simulink model "test9_1"  (R2024a)
settings: Solver=FixedStepAuto  StartTime=0.0  StopTime=20  FixedStep=0.001  MaxStep=1e-2  RelTol=1e-3
libraries: fl_lib x14, nesl_utility x12, simulink x5, sdl_lib x4
settings Model: DataDictionary=test4.sldd  Creator=18311  LastModifiedBy=18311

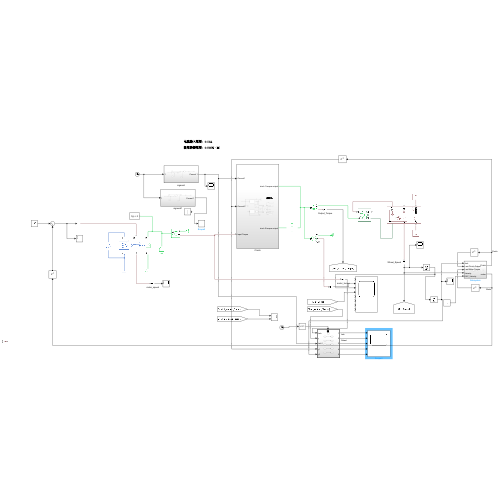
[thumbnail: Simulink's stored preview of the top-level diagram]
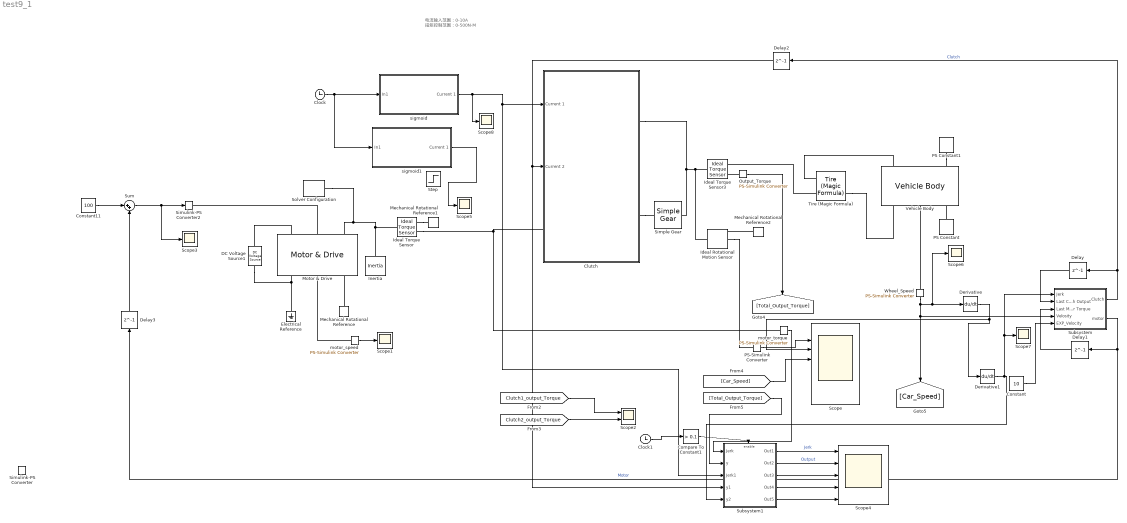
== system test9_1 ==
  note: 电流输入范围：0-10A
      | 扭矩控制范围：0-500N·M
  Clock : Clock
  Clock1 : Clock
  Clutch : Subsystem
  Compare To Constant1 : simulink/Logic and Bit Operations/Compare To Constant  relop=>  const=0.1  OutDataTypeStr=boolean
  Constant : Constant  Value=10
  Constant11 : Constant  Value=100
  DC Voltage Source1 : fl_lib/Electrical/Electrical Sources/DC Voltage Source  v0=220 V
  Delay{,1..3} (4 alike) : Delay  DelayLength=1  InitialCondition=0
  Derivative : Derivative
  Derivative1 : Derivative
  Electrical Reference : fl_lib/Electrical/Electrical Elements/Electrical Reference
  Ideal Rotational Motion Sensor : fl_lib/Mechanical/Mechanical Sensors/Ideal Rotational Motion Sensor  reference=foundation.enum.MeasurementReference.difference  acceleration_port=false  velocity_port=true  position_port=true  wrap_angle=false  offset=0 rad
  Ideal Torque Sensor : fl_lib/Mechanical/Mechanical Sensors/Ideal Torque Sensor
  Ideal Torque Sensor3 : fl_lib/Mechanical/Mechanical Sensors/Ideal Torque Sensor
  Inertia : fl_lib/Mechanical/Rotational Elements/Inertia  inertia=0.01 kg*m^2  num_ports=foundation.enum.numPorts2.one  w_specify=off  w_priority=High  w=0 rad/s  w_nominal_specify=off  w_nominal_value=1  w_nominal_unit=rad/s  t_specify=off  t_priority=None  t=0 N*m  t_nominal_specify=off  t_nominal_value=1  t_nominal_unit=N*m
  Mechanical Rotational Reference : fl_lib/Mechanical/Rotational Elements/Mechanical Rotational Reference
  Mechanical Rotational Reference1 : fl_lib/Mechanical/Rotational Elements/Mechanical Rotational Reference
  Mechanical Rotational Reference2 : fl_lib/Mechanical/Rotational Elements/Mechanical Rotational Reference
  Motor & Drive : sdl_lib/Engines & Motors/Motor & Drive  torque_max=500 N*m  power_max=450 kW  Tc=1 s  eff=75  w_eff=100 rpm  T_eff=400 N*m  thermal_port=simscape.enum.thermaleffects.omit  thermal_mass=100 J/K  temperature_specify=off  temperature_priority=High  temperature=300 K  temperature_nominal_specify=off  temperature_nominal_value=1  temperature_nominal_unit=K
      settings: InternalSimscapePortConfiguration="{\"Bottom\":[],\"Left\":[{\"id\":\"Vp\",\"label\":\"+\",\"type\":\"foundation.electrical.electrical\"},{\"id\":\"Tr\",\"label\":\"Tr\",\"type\":\"input\"},{\"id\":\"R\",\"label\":\"R\",\"type\":\"foundation.mechanical.rotational.rotational\"}],\"Right\":[{\"id\":\"Vm\",\"label\":\"-\",\"type\":\"foundation.electrical.electrical\"},{\"id\":\"Omega\",\"label\":\"w\",\"type\":\"output\"},{\"id\":\"C\",\"label\":\"C\",\"type\":\"foundation.mechanical.rotational.rotational\"}],\"Top\":[]}"
  Output_Torque : nesl_utility/PS-Simulink Converter  PhysicalDomain=network_engine_domain  SubClassName=ps_output  LeftPortType=input  RightPortType=output  PseudoPeriodic=off  Frequencies=[]  VectorFormat=inherit  Unit=inherit  AffineConversion=off
  PS Constant : fl_lib/Physical Signals/Sources/PS Constant  constant=0
  PS Constant1 : fl_lib/Physical Signals/Sources/PS Constant  constant=0
  PS-Simulink Converter : nesl_utility/PS-Simulink Converter  PhysicalDomain=network_engine_domain  SubClassName=ps_output  LeftPortType=input  RightPortType=output  PseudoPeriodic=off  Frequencies=[]  VectorFormat=inherit  Unit=inherit  AffineConversion=off
  Scope : Scope  NumInputPorts=8
  Scope{1,3,5..8} (6 alike) : Scope
  Scope2 : Scope  NumInputPorts=2
  Scope4 : Scope  NumInputPorts=5
  Simple Gear : sdl_lib/Gears/Simple Gear  ratio=1.5  rotation_direction=sdl.enum.shaftOutputDirection.same  enable_faults=simscape.enum.onoff.off  efficiency_fault=0.05  fault_angles=pi / 12 rad  friction_model=sdl.enum.gear_efficiencies_load.off  T_noload=0.1 N*m  T_nom=5 N*m  efficiency_nom=0.8  efficiency=0.8  temperature_TLU=[280, 300, 320] K  load_TLU=[1, 5, 10] N*m  efficiency_TLU=[.95, .9, .85]  efficiency_TLU2=[.85, .8, .75; .95, .9, .85; .85, .8, .7]  w_thr=0.01 rad/s  pwr_thr=0.001 W  enable_backlash=false  hardstop_model=simscape.enum.hardstop.smooth  backlash_distance=1e-3 mm  r_base=0.1 m  transition=1e-4 mm  backlash_stiffness=1e6 N/m  backlash_damping=1e3 N*s/m  coeff_rest=0.7  v_tol=0.001 m/s  f_tol=0.001 N  mu_visc=[0, 0] N*m*s/rad  thermal_mass=50 J/K  temperature_specify=off  temperature_priority=High  temperature=300 K  temperature_nominal_specify=off  temperature_nominal_value=1  temperature_nominal_unit=K  x_backlash_specify=off  x_backlash_priority=None  x_backlash=0 mm  x_backlash_nominal_specify=off  x_backlash_nominal_value=1  x_backlash_nominal_unit=mm  f_hardstop_specify=off  f_hardstop_priority=None  f_hardstop=0 N  f_hardstop_nominal_specify=off  f_hardstop_nominal_value=1  f_hardstop_nominal_unit=N  v_backlash_specify=off  v_backlash_priority=None  v_backlash=0 m/s  v_backlash_nominal_specify=off  v_backlash_nominal_value=1  v_backlash_nominal_unit=m/s
  Simulink-PS Converter : nesl_utility/Simulink-PS Converter  PhysicalDomain=network_engine_domain  SubClassName=ps_input  LeftPortType=input  RightPortType=output  PseudoPeriodic=off  Frequencies=[]  NoiseDistribution=none  NoiseParameters=[]  Unit=1  AffineConversion=off  FilteringAndDerivatives=provide  SimscapeFilterOrder=1  InputFilterTimeConstant=0.001  UdotUserProvided=0
  Simulink-PS Converter2 : nesl_utility/Simulink-PS Converter  PhysicalDomain=network_engine_domain  SubClassName=ps_input  LeftPortType=input  RightPortType=output  PseudoPeriodic=off  Frequencies=[]  NoiseDistribution=none  NoiseParameters=[]  Unit=1  AffineConversion=off  FilteringAndDerivatives=provide  SimscapeFilterOrder=1  InputFilterTimeConstant=0.001  UdotUserProvided=0
  Solver Configuration : nesl_utility/Solver Configuration  PhysicalDomain=network_engine_domain  SubClassName=solver  LeftPortType=input  RightPortType=generic  Tones=[]  Harmonics=[]  SimulateNoise=off  Profile=off  UseLocalSampling=off  EnableSwitchedLinearOptims=on  FrequencyDomain=off  UseCCode=off  RelTol=0.001  AbsTol=0.001  MinStep=1e-09  ToWorkspace=off  RevertToSquareIcSolve=off  NumHomotopyIterations=100  PhasorMode=off  PhasorModeNumHarmonics=1  ConsistencySolver=NEWTON_XTOL_AFTER_FTOL  IndexReductionMethod=DerivativeReplacement  DoDC=off  ResidualTolerance=1e-09  ConsistencyTolSource=GLOBAL  ConsistencyAbsTol=0.001  ConsistencyRelTol=0.001  ConsistencyTolFactor=0.001  UseLocalSolver=off  LocalSolverChoice=NE_BACKWARD_EULER_ADVANCER  ResolveIndetEquations=on  FunctionEvalNumThread=1  LocalSolverSampleTime=0.001  DoFixedCost=off  MaxNonlinIter=3  MaxModeIter=2  ComputeImpulses=off  ImpulseIterations=2  LinearAlgebra=auto  LinearAlgebraNumThread=0  EquationFormulation=NE_TIME_EF  DelaysMemoryBudget=1024  AutomaticFiltering=on  FilteringTimeConstant=0.001  PartitionStorageMethod=AS_NEEDED  PartitionMemoryBudget=1024  PartitionMethod=ROBUST  MultibodyUseLocalSolver=off  MultibodyLocalSolverChoice=ODE1  MultibodyLocalSolverSampleTime=0.001
  Step : Step  Time=5  After=10  SampleTime=0
  Subsystem : Subsystem
  Subsystem1 : Subsystem
  Sum : Sum  Inputs=|++
  Tire (Magic Formula) : sdl_lib/Tires & Vehicles/Tire (Magic Formula)  parameterization=sdl.enum.magic_tire_model.peak  F_z1=200 N  F_x1=250 N  kappa1=10  B_m=10  C_m=1.9  D_m=1  E_m=0.97  fz0=4000 N  p_Cx=1.685  p_Dx=[1.21, -.037]  p_Ex=[.344, .095, -.02, 0]  p_Kx=[21.51, -.163, .245]  p_Hx=[-.002, .002]  p_Vx=[0, 0]  rolling_radius_model=sdl.enum.RollingRadiusParameterization.Constant  r_e=0.3 m  r_0=0.3 m  breff=8.39  dreff=0.26  freff=0.074  q_re0=0.99  q_v1=0.008  longvl=17 m/s  cz=5e5 N/m  model_resistance=false  resistance_model=sdl.enum.rollingResistanceParameterization.constant  coeff=0.015  p_tire=250e3 Pa  alpha=-0.003  beta=0.97  coeff_a=84e-4  coeff_b=6.2e-4 s/m  coeff_c=1.6e-4 s^2/m^2  p_tire0=240e3 Pa  fz0_resistance=4000 N  vH0=16 m/s  q_Sy=[.0082, 0, .0014, .001, 0, 0, 1.08, -.5]  v_thr=0.001 m/s  enable_scaling_coefficients=false  lfzO=1  lcx=1  lmux=1  lex=1  lkx=1  lhx=1  lvx=1  lmy=1  model_compliance=sdl.enum.compliance.off  stiffness=1e6 N/m  damping=1000 N*s/m  model_inertia=sdl.enum.model_inertia.off  inertia=1 kg*m^2  initial_velocity=0 rad/s  vxlow=1 m/s  v_tr_thr=0.1 m/s  kpumin=-1.5  kpumax=1.5
  Vehicle Body : sdl_lib/Tires & Vehicles/Vehicle Body  mass=300 kg  n_w=1  x_f=1.4 m  x_r=1.6 m  y_c=0.5 m  mass_var=simscape.enum.onoff.off  g=9.81 m/s^2  liftoff_warning=simscape.enum.onoff.off  area=3 m^2  Cd=0.4  rho=1.18 kg/m^3  model_pitch=simscape.enum.onoff.off  inertia=4000 kg*m^2  suspension_model=sdl.enum.linearTLU.linear  k_f=1e4 N/m  b_f=1e4 N*s/m  k_r=1e4 N/m  b_r=1e4 N*s/m  k_f_TLU=[-2000, -1000, 0, 1000, 2000] N  x_f_TLU=[-.4, -.2, 0, .2, .4] m  b_f_TLU=[-200, -100, 0, 100, 200] N  v_f_TLU=[-4, -2, 0, 2, 4] m/s  k_r_TLU=[-2000, -1000, 0, 1000, 2000] N  x_r_TLU=[-.4, -.2, 0, .2, .4] m  b_r_TLU=[-200, -100, 0, 100, 200] N  v_r_TLU=[-4, -2, 0, 2, 4] m/s  interp_method=simscape.enum.interpolation.linear  extrap_method=simscape.enum.extrapolation.linear  model_hardstop=simscape.enum.onoff.off  upper_bound_f=.25 m  lower_bound_f=-.25 m  stop_k_f=1e6 N/m  stop_b_f=150 N*s/m  upper_bound_r=.25 m  lower_bound_r=-.25 m  stop_k_r=1e6 N/m  stop_b_r=150 N*s/m  initial_pitch=0 rad  initial_pitch_rate=0 rad/s  v_specify=off  v_priority=High  v=0 m/s  v_nominal_specify=off  v_nominal_value=1  v_nominal_unit=m/s
  Wheel_Speed : nesl_utility/PS-Simulink Converter  PhysicalDomain=network_engine_domain  SubClassName=ps_output  LeftPortType=input  RightPortType=output  PseudoPeriodic=off  Frequencies=[]  VectorFormat=inherit  Unit=inherit  AffineConversion=off
  motor_speed : nesl_utility/PS-Simulink Converter  PhysicalDomain=network_engine_domain  SubClassName=ps_output  LeftPortType=input  RightPortType=output  PseudoPeriodic=off  Frequencies=[]  VectorFormat=inherit  Unit=inherit  AffineConversion=off
  motor_torque : nesl_utility/PS-Simulink Converter  PhysicalDomain=network_engine_domain  SubClassName=ps_output  LeftPortType=input  RightPortType=output  PseudoPeriodic=off  Frequencies=[]  VectorFormat=inherit  Unit=inherit  AffineConversion=off
  sigmoid : Subsystem
  sigmoid1 : Subsystem
  wires:
  motor_torque/1 -> Subsystem1/1(Jerk)
  motor_speed/1 -> Scope1/1
  Wheel_Speed/1 -> [Car_Speed], Subsystem/4(Velosity), Scope6/1, Derivative/1
  [Total_Output_Torque] -> Subsystem1/2(y)
  [Car_Speed] -> Scope/4
  Output_Torque/1 -> [Total_Output_Torque]
  PS-Simulink Converter/1 -> Scope/2
  Derivative/1 -> Derivative1/1, Scope/3
  Constant11/1 -> Sum/1
  Sum/1 -> Scope3/1, Simulink-PS Converter2/1
  Subsystem/2(motor) -> Delay3/1, Delay1/1  "Motor"
  Delay3/1 -> Sum/2
  Subsystem/1(Clutch) -> Delay2/1, Delay/1  "Clutch"
  [Clutch1_output_Torque] -> Scope2/1
  [Clutch2_output_Torque] -> Scope2/2
  Derivative1/1 -> Subsystem1/5(y2), Scope7/1, Subsystem/1(Jerk)
  sigmoid/1(Current 1) -> Scope8/1, Subsystem1/3(Jerk1), Clutch/1(Current 1)
  Clock/1 -> sigmoid1/1(In1), sigmoid/1(In1)
  Constant/1 -> Subsystem/5(EXP_Velocity)
  Delay/1 -> Subsystem/2(Last Clutch Output)
  Delay1/1 -> Subsystem/3(Last Motor Torque)
  Delay2/1 -> Subsystem1/4(y1), Clutch/2(Current 2)
  Clock1/1 -> Compare To Constant1/1
  Compare To Constant1/1 -> Subsystem1/Enable
  Subsystem1/1(Out1) -> Scope4/1  "Jerk"
  Subsystem1/2(Out2) -> Scope4/2  "Output"
  Subsystem1/3(Out3) -> Scope4/3
  Subsystem1/4(Out4) -> Scope4/4
  Subsystem1/5(Out5) -> Scope4/5
  sigmoid1/1(Current 1) -> Scope5/1
  connections:
  Motor & Drive/LConn1 -- DC Voltage Source1/LConn1
  Electrical Reference/LConn1 -- DC Voltage Source1/RConn1 -- Motor & Drive/RConn1
  Mechanical Rotational Reference/LConn1 -- Motor & Drive/RConn3
  Inertia/LConn1 -- Solver Configuration/RConn1 -- Motor & Drive/LConn3 -- Ideal Torque Sensor/LConn1
  Tire (Magic Formula)/RConn2 -- Vehicle Body/LConn1
  Vehicle Body/RConn1 -- Tire (Magic Formula)/LConn1
  PS Constant/RConn1 -- Vehicle Body/LConn3
  PS Constant1/RConn1 -- Vehicle Body/RConn3
  Ideal Torque Sensor3/LConn1 -- Ideal Rotational Motion Sensor/LConn1 -- Clutch/RConn1 -- Simple Gear/RConn1
  Ideal Torque Sensor/RConn2 -- motor_torque/LConn1 -- Clutch/LConn1
  Wheel_Speed/LConn1 -- Vehicle Body/LConn2
  motor_speed/LConn1 -- Motor & Drive/RConn2
  Output_Torque/LConn1 -- Ideal Torque Sensor3/RConn2
  Ideal Torque Sensor/RConn1 -- Mechanical Rotational Reference1/LConn1
  Clutch/RConn2 -- Simple Gear/LConn1
  Motor & Drive/LConn2 -- Simulink-PS Converter2/RConn1
  Mechanical Rotational Reference2/LConn1 -- Ideal Rotational Motion Sensor/RConn1
  Ideal Rotational Motion Sensor/RConn2 -- PS-Simulink Converter/LConn1
  Tire (Magic Formula)/LConn2 -- Ideal Torque Sensor3/RConn1

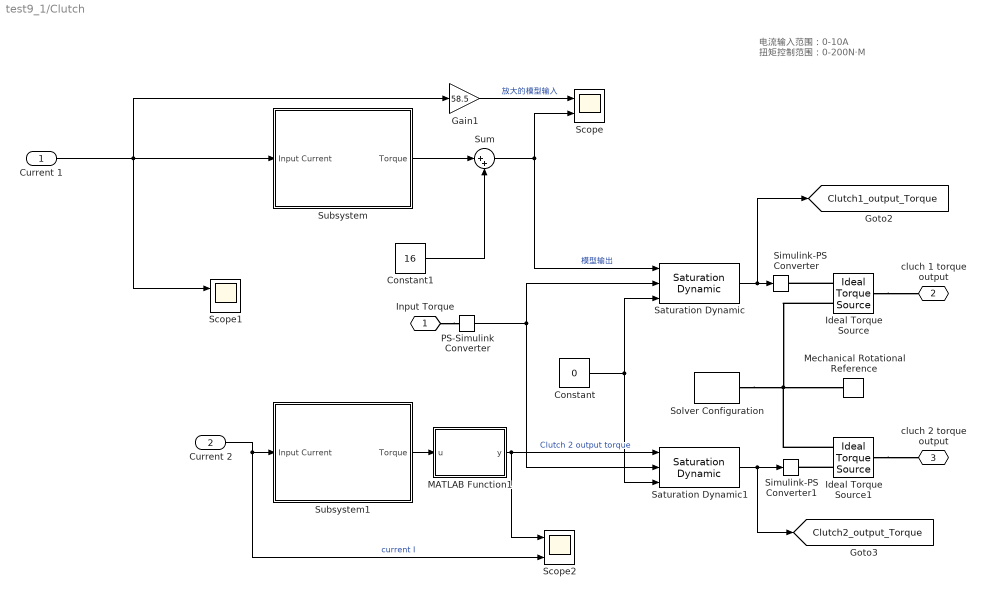
== system test9_1/Clutch ==
  note: 电流输入范围：0-10A
      | 扭矩控制范围：0-200N·M
  Current 1 : Inport
  Current 2 : Inport  Port=2
  Constant : Constant  Value=0
  Constant1 : Constant  Value=16
  Gain1 : Gain  Gain=58.5
  Ideal Torque Source : fl_lib/Mechanical/Mechanical Sources/Ideal Torque Source
  Ideal Torque Source1 : fl_lib/Mechanical/Mechanical Sources/Ideal Torque Source
  MATLAB Function1 : MATLAB Function  TreatAsAtomicUnit=on
  Mechanical Rotational Reference : fl_lib/Mechanical/Rotational Elements/Mechanical Rotational Reference
  PS-Simulink Converter : nesl_utility/PS-Simulink Converter  PhysicalDomain=network_engine_domain  SubClassName=ps_output  LeftPortType=input  RightPortType=output  PseudoPeriodic=off  Frequencies=[]  VectorFormat=inherit  Unit=inherit  AffineConversion=off
  Saturation Dynamic : simulink/Discontinuities/Saturation Dynamic  OutMin=[]  OutMax=[]  OutDataTypeStr=Inherit: Same as second input  OutDataType=fixdt(1, 16)  OutScaling=2^-10  DoSatur=off
  Saturation Dynamic1 : simulink/Discontinuities/Saturation Dynamic  OutMin=[0]  OutMax=[]  OutDataTypeStr=Inherit: Same as second input  OutDataType=fixdt(1, 16)  OutScaling=2^-10  DoSatur=off
  Scope : Scope  NumInputPorts=2
  Scope1 : Scope  NumInputPorts=2
  Scope2 : Scope  NumInputPorts=3
  Simulink-PS Converter : nesl_utility/Simulink-PS Converter  PhysicalDomain=network_engine_domain  SubClassName=ps_input  LeftPortType=input  RightPortType=output  PseudoPeriodic=off  Frequencies=[]  NoiseDistribution=none  NoiseParameters=[]  Unit=1  AffineConversion=off  FilteringAndDerivatives=provide  SimscapeFilterOrder=1  InputFilterTimeConstant=0.001  UdotUserProvided=0
  Simulink-PS Converter1 : nesl_utility/Simulink-PS Converter  PhysicalDomain=network_engine_domain  SubClassName=ps_input  LeftPortType=input  RightPortType=output  PseudoPeriodic=off  Frequencies=[]  NoiseDistribution=none  NoiseParameters=[]  Unit=1  AffineConversion=off  FilteringAndDerivatives=provide  SimscapeFilterOrder=1  InputFilterTimeConstant=0.001  UdotUserProvided=0
  Solver Configuration : nesl_utility/Solver Configuration  PhysicalDomain=network_engine_domain  SubClassName=solver  LeftPortType=input  RightPortType=generic  Tones=[]  Harmonics=[]  SimulateNoise=off  Profile=off  UseLocalSampling=off  EnableSwitchedLinearOptims=on  FrequencyDomain=off  UseCCode=off  RelTol=0.001  AbsTol=0.001  MinStep=1e-09  ToWorkspace=off  RevertToSquareIcSolve=off  NumHomotopyIterations=100  PhasorMode=off  PhasorModeNumHarmonics=1  ConsistencySolver=NEWTON_XTOL_AFTER_FTOL  IndexReductionMethod=DerivativeReplacement  DoDC=off  ResidualTolerance=1e-09  ConsistencyTolSource=GLOBAL  ConsistencyAbsTol=0.001  ConsistencyRelTol=0.001  ConsistencyTolFactor=0.001  UseLocalSolver=off  LocalSolverChoice=NE_BACKWARD_EULER_ADVANCER  ResolveIndetEquations=on  FunctionEvalNumThread=1  LocalSolverSampleTime=0.001  DoFixedCost=off  MaxNonlinIter=3  MaxModeIter=2  ComputeImpulses=off  ImpulseIterations=2  LinearAlgebra=auto  LinearAlgebraNumThread=0  EquationFormulation=NE_TIME_EF  DelaysMemoryBudget=1024  AutomaticFiltering=on  FilteringTimeConstant=0.001  PartitionStorageMethod=AS_NEEDED  PartitionMemoryBudget=1024  PartitionMethod=ROBUST  MultibodyUseLocalSolver=off  MultibodyLocalSolverChoice=ODE1  MultibodyLocalSolverSampleTime=0.001
  Subsystem : Subsystem  mask{c=-2, k=58.857, d=0.6, alpha=-37.209}
  Subsystem1 : Subsystem  mask{c=-2, k=58.857, d=0.6, alpha=-37.209}
  Sum : Sum  Inputs=|++
  Input Torque : PMIOPort  Side=Left
  cluch 1 torque output : PMIOPort  Port=2  Side=Right
  cluch 2 torque output : PMIOPort  Port=3  Side=Right
  tag scope: Clutch1_output_Torque=global, Clutch2_output_Torque=global
  wires:
  PS-Simulink Converter/1 -> Saturation Dynamic/2, Saturation Dynamic1/2
  Constant/1 -> Saturation Dynamic/3, Saturation Dynamic1/3
  Saturation Dynamic/1 -> [Clutch1_output_Torque], Simulink-PS Converter/1
  Saturation Dynamic1/1 -> [Clutch2_output_Torque], Simulink-PS Converter1/1
  Current 1/1 -> Subsystem/1(Input Current), Scope1/1, Gain1/1
  Current 2/1 -> Subsystem1/1(Input Current), Scope2/3  "current I"
  Gain1/1 -> Scope/1  "放大的模型输入"
  Subsystem/1(Torque) -> Sum/1
  Sum/1 -> Saturation Dynamic/1, Scope/2  "模型输出"
  Constant1/1 -> Sum/2
  Subsystem1/1(Torque) -> MATLAB Function1/1(u)
  MATLAB Function1/1(y) -> Scope2/1, Saturation Dynamic1/1  "Clutch 2 output torque"
  connections:
  Input Torque/RConn1 -- PS-Simulink Converter/LConn1
  Ideal Torque Source/RConn2 -- Solver Configuration/RConn1 -- Ideal Torque Source1/RConn2 -- Mechanical Rotational Reference/LConn1
  Ideal Torque Source/LConn1 -- cluch 1 torque output/RConn1
  Ideal Torque Source1/LConn1 -- cluch 2 torque output/RConn1
  Ideal Torque Source/RConn1 -- Simulink-PS Converter/RConn1
  Ideal Torque Source1/RConn1 -- Simulink-PS Converter1/RConn1

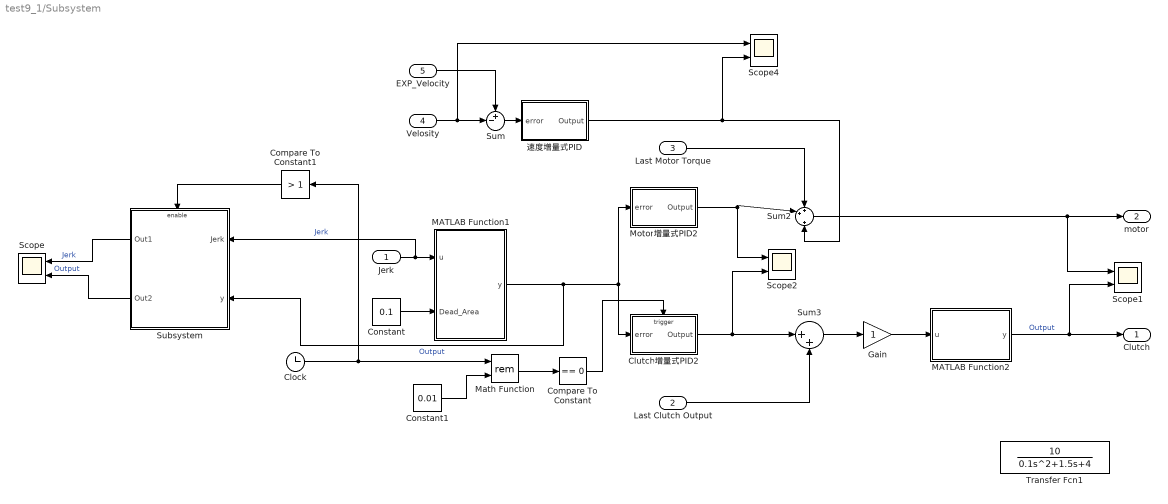
== system test9_1/Subsystem ==
  Jerk : Inport
  Last Clutch Output : Inport  Port=2
  Last Motor Torque : Inport  Port=3
  Velosity : Inport  Port=4
  EXP_Velocity : Inport  Port=5
  Clock : Clock
  Clutch增量式PID2 : Subsystem  mask{Kp=0.09, Ki=0.02, Kd=0.03}
      mask DialogControl ParameterGroupVar Prompt: 参数
  Compare To Constant : simulink/Logic and Bit Operations/Compare To Constant  relop===  const=0  OutDataTypeStr=boolean
  Compare To Constant1 : simulink/Logic and Bit Operations/Compare To Constant  relop=>  const=1  OutDataTypeStr=boolean
  Constant : Constant  Value=0.1
  Constant1 : Constant  Value=0.01
  Gain : Gain
  MATLAB Function1 : MATLAB Function  TreatAsAtomicUnit=on
  MATLAB Function2 : MATLAB Function  TreatAsAtomicUnit=on
  Math Function : Math  Operator=rem
  Motor增量式PID2 : Subsystem  mask{Kp=5, Ki=1, Kd=3}
      mask DialogControl ParameterGroupVar Prompt: 参数
  Scope{,1..2,4} (4 alike) : Scope  NumInputPorts=2
  Subsystem : Subsystem
  Sum : Sum  Inputs=+-|
  Sum2 : Sum  Inputs=++|+
  Sum3 : Sum  Inputs=|++
  Transfer Fcn1 : TransferFcn  Numerator=10  Denominator=[0.1 1.5 4]
  速度增量式PID : Subsystem  mask{Kp=10, Ki=0.001, Kd=1}
      mask DialogControl ParameterGroupVar Prompt: 参数
  Clutch : Outport
  motor : Outport  Port=2
  wires:
  Velosity/1 -> Scope4/1, Sum/2
  EXP_Velocity/1 -> Sum/1
  Jerk/1 -> Subsystem/1(Jerk), MATLAB Function1/1(u)  "Jerk"
  速度增量式PID/1(Output) -> Scope4/2, Sum2/3
  Last Motor Torque/1 -> Sum2/1
  Motor增量式PID2/1(Output) -> Scope2/1, Sum2/2
  Last Clutch Output/1 -> Sum3/2
  Sum/1 -> 速度增量式PID/1(error)
  MATLAB Function1/1(y) -> Subsystem/2(y), Motor增量式PID2/1(error), Clutch增量式PID2/1(error)  "Output"
  Constant/1 -> MATLAB Function1/2(Dead_Area)
  Sum2/1 -> Scope1/1, motor/1
  Sum3/1 -> Gain/1
  Clock/1 -> Compare To Constant1/1, Math Function/1
  Constant1/1 -> Math Function/2
  Math Function/1 -> Compare To Constant/1
  Compare To Constant/1 -> Clutch增量式PID2/Trigger
  Gain/1 -> MATLAB Function2/1(u)
  MATLAB Function2/1(y) -> Scope1/2, Clutch/1  "Output"
  Compare To Constant1/1 -> Subsystem/Enable
  Subsystem/1(Out1) -> Scope/1  "Jerk"
  Subsystem/2(Out2) -> Scope/2  "Output"
  Clutch增量式PID2/1(Output) -> Scope2/2, Sum3/1

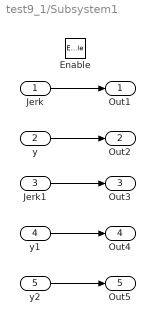
== system test9_1/Subsystem1 ==
  Jerk : Inport
  y : Inport  Port=2
  Jerk1 : Inport  Port=3
  y1 : Inport  Port=4
  y2 : Inport  Port=5
  Enable : EnablePort
  Out1 : Outport
  Out2 : Outport  Port=2
  Out3 : Outport  Port=3
  Out4 : Outport  Port=4
  Out5 : Outport  Port=5
  wires:
  Jerk/1 -> Out1/1
  y/1 -> Out2/1
  Jerk1/1 -> Out3/1
  y1/1 -> Out4/1
  y2/1 -> Out5/1

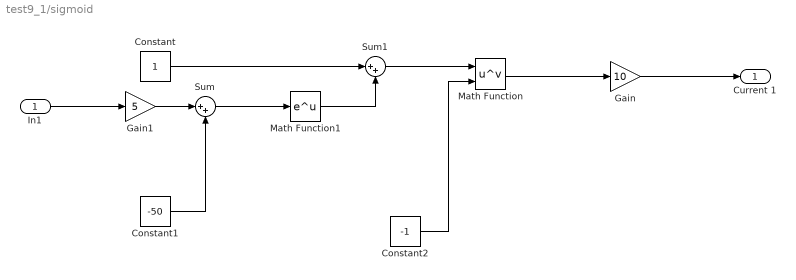
== system test9_1/sigmoid ==
  In1 : Inport
  Constant : Constant
  Constant1 : Constant  Value=-50
  Constant2 : Constant  Value=-1
  Gain : Gain  Gain=10
  Gain1 : Gain  Gain=5
  Math Function : Math  Operator=pow
  Math Function1 : Math
  Sum : Sum  Inputs=|++
  Sum1 : Sum  Inputs=|++
  Current 1 : Outport
  wires:
  Constant1/1 -> Sum/2
  In1/1 -> Gain1/1
  Sum/1 -> Math Function1/1
  Math Function1/1 -> Sum1/2
  Constant/1 -> Sum1/1
  Constant2/1 -> Math Function/2
  Sum1/1 -> Math Function/1
  Math Function/1 -> Gain/1
  Gain/1 -> Current 1/1
  Gain1/1 -> Sum/1

== system test9_1/sigmoid1 ==
  In1 : Inport
  Constant : Constant
  Constant1 : Constant  Value=50
  Constant2 : Constant  Value=-1
  Gain : Gain  Gain=10
  Gain1 : Gain  Gain=5
  Math Function : Math  Operator=pow
  Math Function1 : Math
  Sum : Sum  Inputs=|-+
  Sum1 : Sum  Inputs=|++
  Current 1 : Outport
  wires:
  Constant1/1 -> Sum/2
  In1/1 -> Gain1/1
  Sum/1 -> Math Function1/1
  Math Function1/1 -> Sum1/2
  Constant/1 -> Sum1/1
  Constant2/1 -> Math Function/2
  Sum1/1 -> Math Function/1
  Math Function/1 -> Gain/1
  Gain/1 -> Current 1/1
  Gain1/1 -> Sum/1

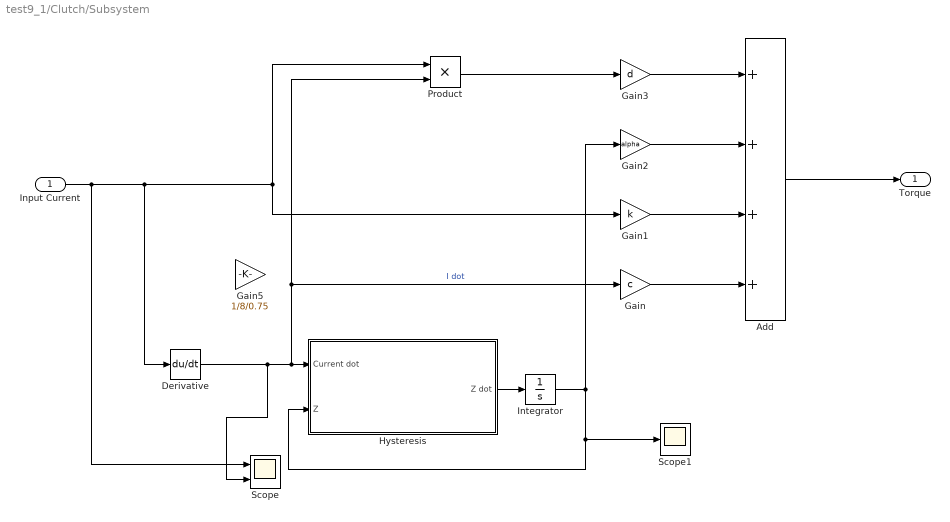
== system test9_1/Clutch/Subsystem ==
  Input Current : Inport
  Add : Sum  Inputs=++++
  Derivative : Derivative
  Gain : Gain  Gain=c
  Gain1 : Gain  Gain=k
  Gain2 : Gain  Gain=alpha
  Gain3 : Gain  Gain=d
  Gain5 : Gain  Gain=1/8/0.75
  Hysteresis : Subsystem  mask{theta=-0.41731, beta=-0.83796, v=2.2221, gamma=2.0211}
  Integrator : Integrator
  Product : Product
  Scope : Scope  NumInputPorts=2
  Scope1 : Scope
  Torque : Outport
  wires:
  Derivative/1 -> Scope/2, Hysteresis/1(Current dot), Product/2, Gain/1  "I dot"
  Gain/1 -> Add/4
  Gain1/1 -> Add/3
  Gain2/1 -> Add/2
  Gain3/1 -> Add/1
  Product/1 -> Gain3/1
  Input Current/1 -> Scope/1, Derivative/1, Product/1, Gain1/1
  Integrator/1 -> Scope1/1, Hysteresis/2(Z), Gain2/1
  Hysteresis/1(Z dot) -> Integrator/1
  Add/1 -> Torque/1

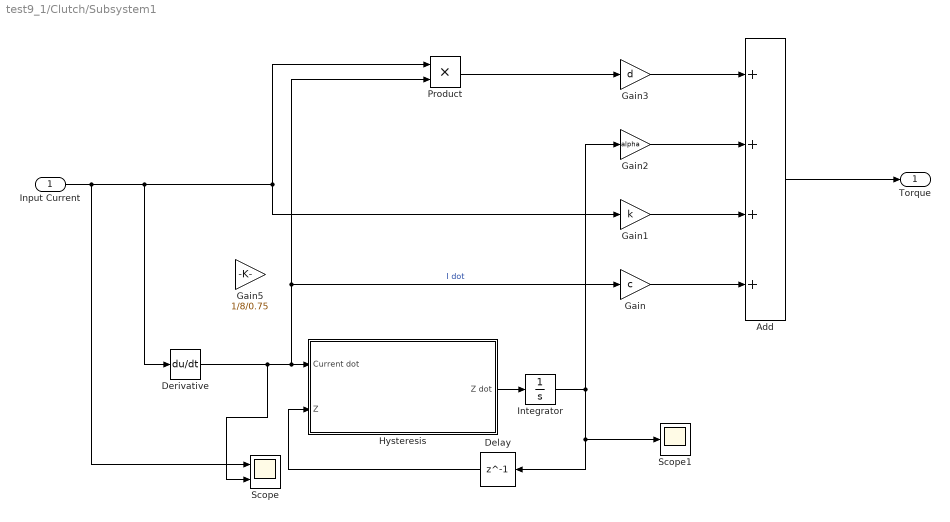
== system test9_1/Clutch/Subsystem1 ==
  Input Current : Inport
  Add : Sum  Inputs=++++
  Delay : Delay  DelayLength=1  InitialCondition=0
  Derivative : Derivative
  Gain : Gain  Gain=c
  Gain1 : Gain  Gain=k
  Gain2 : Gain  Gain=alpha
  Gain3 : Gain  Gain=d
  Gain5 : Gain  Gain=1/8/0.75
  Hysteresis : Subsystem  mask{theta=-0.41731, beta=-0.83796, v=2.2221, gamma=2.0211}
  Integrator : Integrator
  Product : Product
  Scope : Scope  NumInputPorts=2
  Scope1 : Scope
  Torque : Outport
  wires:
  Derivative/1 -> Scope/2, Hysteresis/1(Current dot), Product/2, Gain/1  "I dot"
  Gain/1 -> Add/4
  Gain1/1 -> Add/3
  Gain2/1 -> Add/2
  Gain3/1 -> Add/1
  Product/1 -> Gain3/1
  Input Current/1 -> Scope/1, Derivative/1, Product/1, Gain1/1
  Hysteresis/1(Z dot) -> Integrator/1
  Add/1 -> Torque/1
  Delay/1 -> Hysteresis/2(Z)
  Integrator/1 -> Gain2/1, Scope1/1, Delay/1

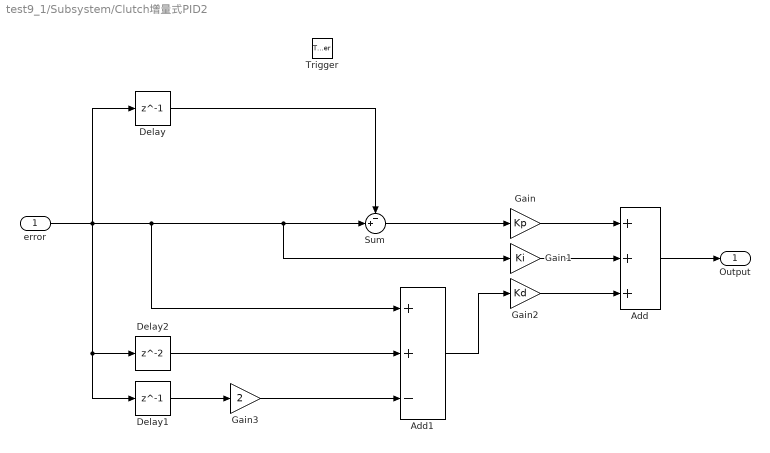
== system test9_1/Subsystem/Clutch增量式PID2 ==
  error : Inport
  Trigger : TriggerPort  VariantControl=(inherit)  PortDimensions=1
  Add : Sum  Inputs=+++
  Add1 : Sum  Inputs=++-
  Delay : Delay  DelayLength=1  InitialCondition=0
  Delay1 : Delay  DelayLength=1  InitialCondition=0
  Delay2 : Delay  InitialCondition=0
  Gain : Gain  Gain=Kp
  Gain1 : Gain  Gain=Ki
  Gain2 : Gain  Gain=Kd
  Gain3 : Gain  Gain=2
  Sum : Sum  Inputs=-+|
  Output : Outport
  wires:
  error/1 -> Delay1/1, Delay2/1, Add1/1, Gain1/1, Sum/2, Delay/1
  Add/1 -> Output/1
  Gain2/1 -> Add/3
  Gain1/1 -> Add/2
  Gain/1 -> Add/1
  Delay/1 -> Sum/1
  Sum/1 -> Gain/1
  Delay1/1 -> Gain3/1
  Gain3/1 -> Add1/3
  Delay2/1 -> Add1/2
  Add1/1 -> Gain2/1

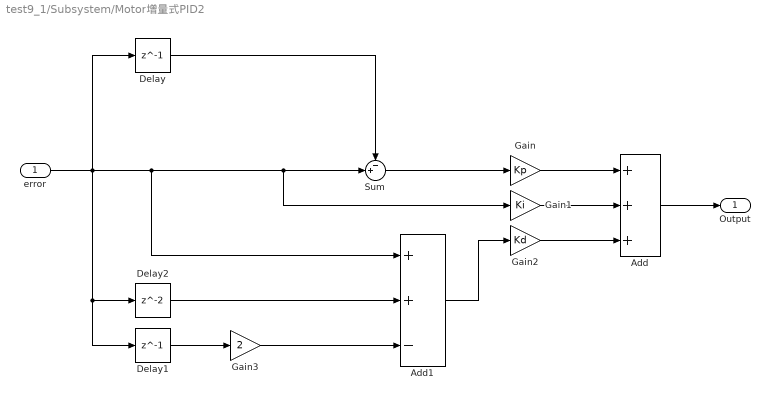
== system test9_1/Subsystem/Motor增量式PID2 ==
  error : Inport
  Add : Sum  Inputs=+++
  Add1 : Sum  Inputs=++-
  Delay : Delay  DelayLength=1  InitialCondition=0
  Delay1 : Delay  DelayLength=1  InitialCondition=0
  Delay2 : Delay  InitialCondition=0
  Gain : Gain  Gain=Kp
  Gain1 : Gain  Gain=Ki
  Gain2 : Gain  Gain=Kd
  Gain3 : Gain  Gain=2
  Sum : Sum  Inputs=-+|
  Output : Outport
  wires:
  error/1 -> Delay1/1, Delay2/1, Add1/1, Gain1/1, Sum/2, Delay/1
  Add/1 -> Output/1
  Gain2/1 -> Add/3
  Gain1/1 -> Add/2
  Gain/1 -> Add/1
  Delay/1 -> Sum/1
  Sum/1 -> Gain/1
  Delay1/1 -> Gain3/1
  Gain3/1 -> Add1/3
  Delay2/1 -> Add1/2
  Add1/1 -> Gain2/1

== system test9_1/Subsystem/Subsystem ==
  Jerk : Inport
  y : Inport  Port=2
  Enable : EnablePort
  Out1 : Outport
  Out2 : Outport  Port=2
  wires:
  Jerk/1 -> Out1/1
  y/1 -> Out2/1

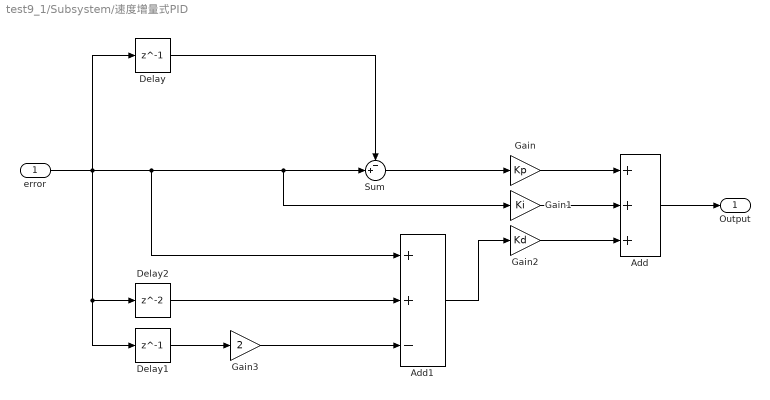
== system test9_1/Subsystem/速度增量式PID ==
  error : Inport
  Add : Sum  Inputs=+++
  Add1 : Sum  Inputs=++-
  Delay : Delay  DelayLength=1  InitialCondition=0
  Delay1 : Delay  DelayLength=1  InitialCondition=0
  Delay2 : Delay  InitialCondition=0
  Gain : Gain  Gain=Kp
  Gain1 : Gain  Gain=Ki
  Gain2 : Gain  Gain=Kd
  Gain3 : Gain  Gain=2
  Sum : Sum  Inputs=-+|
  Output : Outport
  wires:
  error/1 -> Delay1/1, Delay2/1, Add1/1, Gain1/1, Sum/2, Delay/1
  Add/1 -> Output/1
  Gain2/1 -> Add/3
  Gain1/1 -> Add/2
  Gain/1 -> Add/1
  Delay/1 -> Sum/1
  Sum/1 -> Gain/1
  Delay1/1 -> Gain3/1
  Gain3/1 -> Add1/3
  Delay2/1 -> Add1/2
  Add1/1 -> Gain2/1

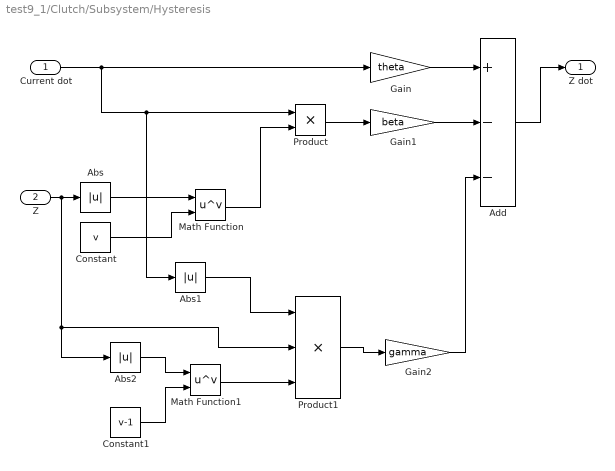
== system test9_1/Clutch/Subsystem/Hysteresis ==
  Current dot : Inport
  Z : Inport  Port=2
  Abs : Abs  SaturateOnIntegerOverflow=off
  Abs1 : Abs  SaturateOnIntegerOverflow=off
  Abs2 : Abs  SaturateOnIntegerOverflow=off
  Add : Sum  Inputs=+--
  Constant : Constant  Value=v
  Constant1 : Constant  Value=v-1
  Gain : Gain  Gain=theta
  Gain1 : Gain  Gain=beta
  Gain2 : Gain  Gain=gamma
  Math Function : Math  Operator=pow
  Math Function1 : Math  Operator=pow
  Product : Product
  Product1 : Product  Inputs=3
  Z dot : Outport
  wires:
  Current dot/1 -> Abs1/1, Product/1, Gain/1
  Gain/1 -> Add/1
  Z/1 -> Product1/2, Abs2/1, Abs/1
  Math Function/1 -> Product/2
  Product/1 -> Gain1/1
  Gain1/1 -> Add/2
  Math Function1/1 -> Product1/3
  Abs1/1 -> Product1/1
  Add/1 -> Z dot/1
  Abs/1 -> Math Function/1
  Constant/1 -> Math Function/2
  Product1/1 -> Gain2/1
  Gain2/1 -> Add/3
  Abs2/1 -> Math Function1/1
  Constant1/1 -> Math Function1/2

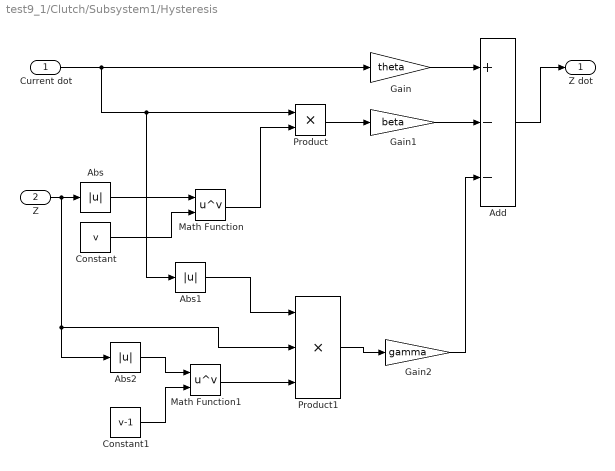
== system test9_1/Clutch/Subsystem1/Hysteresis ==
  Current dot : Inport
  Z : Inport  Port=2
  Abs : Abs  SaturateOnIntegerOverflow=off
  Abs1 : Abs  SaturateOnIntegerOverflow=off
  Abs2 : Abs  SaturateOnIntegerOverflow=off
  Add : Sum  Inputs=+--
  Constant : Constant  Value=v
  Constant1 : Constant  Value=v-1
  Gain : Gain  Gain=theta
  Gain1 : Gain  Gain=beta
  Gain2 : Gain  Gain=gamma
  Math Function : Math  Operator=pow
  Math Function1 : Math  Operator=pow
  Product : Product
  Product1 : Product  Inputs=3
  Z dot : Outport
  wires:
  Current dot/1 -> Abs1/1, Product/1, Gain/1
  Gain/1 -> Add/1
  Z/1 -> Product1/2, Abs2/1, Abs/1
  Math Function/1 -> Product/2
  Product/1 -> Gain1/1
  Gain1/1 -> Add/2
  Math Function1/1 -> Product1/3
  Abs1/1 -> Product1/1
  Add/1 -> Z dot/1
  Abs/1 -> Math Function/1
  Constant/1 -> Math Function/2
  Product1/1 -> Gain2/1
  Gain2/1 -> Add/3
  Abs2/1 -> Math Function1/1
  Constant1/1 -> Math Function1/2

== matlab function test9_1/Subsystem/MATLAB Function2 ==
  data: u input; y output
function y = fcn(u)

if u < 0
    y = 0;
elseif u> 10
    y = 10;
else
    y = u;
end

== matlab function test9_1/Clutch/MATLAB Function1 ==
  data: u input; y output
function y = fcn(u)

if u<0
    y = 0;
else
    y = u;
end

== matlab function test9_1/Subsystem/MATLAB Function1 ==
  data: u input; y output; Dead_Area input
function y = fcn(u,Dead_Area)

if (abs(u) >= Dead_Area) && (u< 0)
    y = -1*u ; 
elseif (abs(u) >= Dead_Area) && (u > 0)
       y = -1*u; 
else
 y = 0;
end
